simulink model "Bruening_4t_showshuffle"  (R2015a)
settings: Solver=ode4  SolverMode=MultiTasking  StartTime=0.0  StopTime=inf  FixedStep=BKIN_STEP_TIME  RelTol=1e-3
StartFcn:
  |  warndlg('Dexterit-E models cannot run under simulation. Please compile your model and run it from within Dexterit-E.');set_param(bdroot,'SimulationCommand','stop')
model workspace (MAT data in the model file):
  BKIN_STEP_TIME = 0.00025
  col_x = 1
  col_y = 2
  E_TARGET_ON = 3
  E_HOLD_AT_TARGET = 5
  LOGICAL_RADIUS = 4
  START_TARGET_COL = 1
  END_TARGET_COL = 2
  ROTATION_CENTER = 5
  WAIT_AT_1stTARGET_COL = 7
  MAXREACHTIME_COL = 8
  DELAY_POSTTRIAL_COL = 9
  E_STAY_CENTER = 2
  VISUAL_RADIUS = 3
  COLOR = 5
  ALTCOLOR = 6
  STROKECOLOUR = 7
  STROKEWIDTH = 9
  TARGET_EGG = 6
  LABEL_TEXT = 12
  LABEL_COLOUR = 13
  LABEL_HEIGHT = 14
  TEXT_DISPLAY_TARGET = 10
  ALTSTROKECOLOUR = 8
  SEGMENT_COUNT = 11
  E_TARGET_MISS = 6
  END_X = 10
  END_Y = 11
  E_LEFT_RING = 4
  E_START_BLOCK = 10
  BKIN_KINEMATIC_FRAME_SIZE = 400
  E_NO_EVENT = 1
  TARGET_IN_USE = 3
  R_PROB = 4
  E_R_TARG1 = 7
  E_M_TARG1 = 12
  E_R_TARG2 = 8
  E_M_TARG2 = 13
  E_R_TARG3 = 9
  E_M_TARG3 = 14
  E_R_TARG4 = 11
  E_M_TARG4 = 15
  WAIT_TIME = 12
  TONE_DURATION = 13
  FLASH_INTER = 14
  FLASH_NUM = 15
  BREAK_T1 = 16
  BREAK_T2 = 17
  ALTVISUAL_RADIUS = 15
  ALTCOLOR2 = 16
undefined symbols (not defined in the file or in its folder): slselsubs
libraries: Video x15, simulink x12, xpcrtudplib x12, xpcutilitieslib x10, xpcobsoletelib x8, ethercat x2, General x2, slrtlib x2, KINARM_general x1
(part 1 of 6)
CloseFcn:
  | rtwprivate ssgencode ModelCloseRequest b2lab2d
settings Model: ModifiedComment=chris -- Wed Feb 16 09:18:30 2005 -- Version 1.1384  ModifiedHistory=Feb 16/05 - Add error repeat, add offset ramp  CovHTMLOptions=-sRT=1 -sVT=0 -aTS=1 -bRG=1 -bTC=1 -hTR=0 -nFC=0 -scm=1 -bcm=1 -xEv=0  ExtModeArmWhenConnect=off  ExtModeLogAll=off  Creator=Chris Grebeldinger  LastModifiedBy=User
settings SolverCC: EnableConcurrentExecution=on  AutoInsertRateTranBlk=on
settings DataIOCC: LimitDataPoints=off  SignalLoggingSaveFormat=ModelDataLogs  SaveOutput=off  SaveTime=off  SignalLoggingName=sigsOut
settings OptimizationCC: BlockReduction=off  BooleanDataType=off  OptimizeBlockIOStorage=off  BufferReuse=off  GlobalBufferReuse=off  ExpressionFolding=off  ExpressionDepthLimit=2147483647  LocalBlockOutputs=off  InitFltsAndDblsToZero=on
settings DebuggingCC: SaveWithParameterizedLinksMsg=none  UnderspecifiedInitializationDetection=Classic  MergeDetectMultiDrivingBlocksExec=none  SignalResolutionControl=TryResolveAll  MultiTaskDSMMsg=warning  FcnCallInpInsideContextMsg=UseLocalSettings  StateNameClashWarn=warning  StrictBusMsg=ErrorOnBusTreatedAsVector
settings HardwareCC: ProdIntDivRoundTo=Zero  ProdEndianess=LittleEndian  ProdLongLongMode=on  ProdHWDeviceType=Generic->32-bit x86 compatible  TargetHWDeviceType=32-bit Generic
settings SFSimCC: SimParseCustomCode=off
settings RTWCC: SystemTargetFile=slrt.tlc  TemplateMakefile=slrt_default_tmf  Description=Simulink Real-Time  RTWCompilerOptimization=on
settings CodeAppCC: MaxIdLength=63
settings SimulinkRealTimeCC: TargetFcnLib=ansi_tfl_tmw.mat  GeneratePreprocessorConditionals=Disable all  xPCisDownloadable=off
settings ConfigComp: Description=Design Verifier Custom Configuration Component  DVMaxTestCaseSteps=500  DVTestSuiteOptimization=CombinedObjectives (Nonlinear Extended)

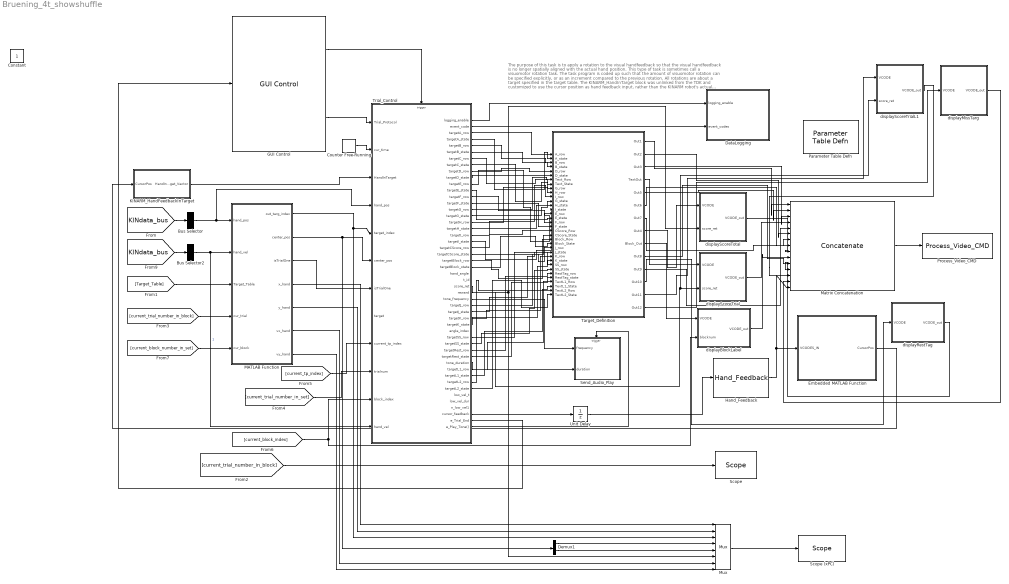
== system Bruening_4t_showshuffle ==
  note: The purpose of this task is to apply a rotation to the visual handfeedback so that the visual handfeedback is no longer spatially aligned with the actual hand position.
      | This type of task is sometimes call a visuomotor rotation task.
      | The task program is coded up such that the amount of visuomotor rotation can be specified explicitly, or as an increment compared to the previous rotation.
      | All rotations are about a target specified in the target table.
      |
      | The KINARM_HandInTarget block was unlinked from the TDK and customized to use the cursor position as hand feedback input, rather than the KINARM robot's actual location.
  Bus Selector : BusSelector  OutputSignals=Robot1.a1_hand_position  OutputAsBus=on
  Bus Selector2 : BusSelector  OutputSignals=Robot1.a1_hand_velocities  OutputAsBus=on
  Counter Free-Running : simulink/Sources/Counter Free-Running  NumBits=32  tsamp=.001
  DataLogging : Subsystem  AncestorBlock=General/DataLogging  mask(DataLogging){log_event_codes=on, log_analog_inputs=off}
      mask prompts: log_event_codes "Log event codes"; log_analog_inputs "Log analog inputs"
      mask help:
      | <b>Do not rename this block, it must be called 'DataLogging'.</b>
      | <p>
      | This block collects data and event codes and transfers them to the GUI.
      | <p>
      | This block must be present in all task programs.
      mask init:
      | %this stops us from running a simulation
      | set_param(bdroot,'StartFcn',' warndlg(''Dexterit-E models cannot run under simulation. Please compile your model and run it from within Dexterit-E.'');set_param(bdroot,''SimulationCommand'',''stop'')')
      | 
      | block_path = gcb;  % store block path, as gcb may change with block operations
      |  
      | idxs = findstr(block_path, '/DataLogging');
      | [idxCount, n] = size(idxs);
      | [m, strlen] = size(block_path);
      | bColorSet = 0;
      | 
      | dexcheck();
      | if idxCount == 0 || idxs(1) ~= strlen - 11
      |     fprintf('=========ERROR====================\n');
      |     fprintf('%s should be called DataLogging, attempting to rename.\n', block_path);
      |     try
      |         set_param(block_path, 'Name', 'DataLogging');
      |         block_path = gcb;  % store block path, as gcb may change with block operations
      |         fprintf('Rename successful\n');
      |     catch err
      |         fprintf('Rename failed. You may have 2 DataLogging blocks or another improperly named block.\n');
      |        	set_param(block_path, 'BackgroundColor', '[0.9, 0, 0]');
      |         bColorSet = 1;
      |     end
      |     fprintf('=============================\n');
      | end
      | 
      | log_event_codes = strcmp(get_param(block_path, 'log_event_codes'), 'on');
      | log_analog_inputs = strcmp(get_param(block_path, 'log_analog_inputs'), 'on');
      | 
      | % Handle the event codes setting: swap the 'Event Codes' inport with a constant block or 
      | % vice versa, if necessary, so that it matches the setting.
      | block_type = get_param([block_path '/event_codes'], 'BlockType');
      |  
      | if log_event_codes && ~strcmp(block_type, 'Inport') || ...  % if a change is required...
      |    ~log_event_codes && strcmp(block_type, 'Inport')
      |     
      |     % ...delete the existing block, ...
      |     pos = get_param([block_path '/event_codes'], 'Position');
      |     delete_line(block_path, 'event_codes/1', 'Create Event Codes Subsystem/1');
      |     delete_block([block_path '/event_codes']);
      |     
      |     % ...add an Inport or a 0-value Constant in place of the previous block (according to
      |     % the new setting), update the signal width flag, and then...
      |     if log_event_codes && ~strcmp(block_type, 'Inport')
      |         add_block('built-in/Inport', [block_path '/event_codes'], 'Name', 'event_codes');
      |         set_param([block_path '/Create Event Codes Subsystem/Not Logging Event Codes'], 'Value', '0');
      |     else
      |         add_block('built-in/Constant', [block_path '/event_codes'], 'Name', 'event_codes');
      |         set_param([block_path '/event_codes'], 'Value', '0');
      |         set_param([block_path '/Create Event Codes Subsystem/Not Logging Event Codes'], 'Value', '1');
      |     end
      |     
      |     % ...connect the new block.
      |     set_param([block_path '/event_codes'], 'Position', pos);
      |     add_line(block_path, 'event_codes/1', 'Create Event Codes Subsystem/1');
      | end
      | 
      | % Swap the 'analog_data' inport with a constant block or vice versa according to the corresponding setting.
      | block_type = get_param([block_path '/analog_inputs'], 'BlockType');
      | 
      | if log_analog_inputs && ~strcmp(block_type, 'Inport') || ...  % if a change is required...
      |    ~log_analog_inputs && strcmp(block_type, 'Inport')
      |     
      |     % ...delete the existing block, ...
      |     pos = get_param([block_path '/analog_inputs'], 'Position');
      |     delete_line(block_path, 'analog_inputs/1', 'Create Analog Inputs Subsystem/1');
      |     delete_block([block_path '/analog_inputs']);
      |     
      |     % ...add an Inport or a 0-value Constant in place of the previous block (according to
      |     % the new setting), update the signal width flag, and then...
      |     if log_analog_inputs && ~strcmp(block_type, 'Inport')
      |         add_block('built-in/Inport', [block_path '/analog_inputs'], 'Name', 'analog_inputs');
      |         set_param([block_path '/Create Analog Inputs Subsystem/Not Logging Analog Inputs'], 'Value', '0');
      |     else
      |         add_block('built-in/Constant', [block_path '/analog_inputs'], 'Name', 'analog_inputs');
      |         set_param([block_path '/analog_inputs'], 'Value', '0');
      |         set_param([block_path '/Create Analog Inputs Subsystem/Not Logging Analog Inputs'], 'Value', '1');
      |     end
      |     
      |     % ...connect the new block.
      |     set_param([block_path '/analog_inputs'], 'Position', pos);
      |     add_line(block_path, 'analog_inputs/1', 'Create Analog Inputs Subsystem/1');
      | end
      | 
      | % Create the text label for the block, and use it to create the first in a 
      | % list of drawing commands that will be used to draw the mask icon.
      | label = 'Logging:\n ';
      |  
      | if log_event_codes
      |    label = [label 'Event codes\n'];
      | end
      |  
      | label = [label 'KINARM data\n'];
      |     
      | if log_analog_inputs
      |     label = [label 'Analog inputs\n'];
      | end
      | 
      | draw_commands = 'disp(label); ';
      | 
      | % Ensure the inports appear in a fixed order, and for each inport found add
      | % to the list of drawing commands a command to label it.
      | inports = find_system(block_path, 'LookUnderMasks', 'all', 'FollowLinks', 'on', 'SearchDepth', 1, 'BlockType', 'Inport');
      | 
      | for i = 1:length(inports)
      |     inport_name = char(get_param(inports(i), 'Name'));
      |     
      |     if strcmp(inport_name, 'logging_enable')
      |         port = '1';
      |     elseif strcmp(inport_name, 'event_codes')
      |         port = '2';
      |     elseif strcmp(inport_name, 'analog_inputs') && log_event_codes
      |         port = '3';
      |     elseif strcmp(inport_name, 'analog_inputs')
      |         port = '2';
      |     end
      |     
      |     set_param([block_path '/' inport_name], 'Port', port);
      |     draw_commands = [draw_commands 'port_label(''input'', ' port ', ''' inport_name '''); '];
      | end
      | 
      | % Apply the drawing commands.
      | set_param(block_path, 'MaskDisplay', draw_commands);
      | 
      | %%% Handle background colours if link status changes.  
      | checkBackgroundColour(block_path, 'General');
      | 
      | % For gaze tracking, the packet length is variable, so we need to check off that option the Receive UDP block.
      | set_param([block_path '/Receive_Gaze/Receive'], 'vblLen', 'on')
      | 
      | initPollKINARM();
      mask Help:
      | Sends data and event codes to the GUI.
      | 
      | <H2>Library </H2>
      | General
      | 
      | <H2>Description </H2>
      | <b>Do not rename this block, it must be called 'DataLogging'.</b>
      | <p>
      | The DataLogging block collects data and event codes and sends it to the GUI for saving.  It also passes on Task Program information that is invisible to the user, and so must be present even if no data is going to be saved.
      | <P>
      | <B><I>This block must be present in all Task Programs, even if no data is going to be saved.</I></B>
      | 
      | 
      | <H2>Parameters and Dialog Box</H2>
      | <B>Log event codes: </B> checking this parameter causes the GUI to log event codes specified by the event_codes input.
      | <P>
      | <B>Log analog inputs: </B> checking this parameter causes the GUI to log analog data specified by the analog_inputs input.
      | <P>
      | <B>analog_inputs: </B> this vector input specifies the data from analog inputs and other arbitrary data to be logged by the GUI.
      | <P>
      | <B>event_codes: </B> this input should be a vector of 16 bit integers.  It is passed on to the GUI, which saves the integers as event codes (i.e. they are timestamped so that events that occurred duing a task can be related to the other saved data).
      | <P>
      | <B>logging_enable: </B> this input is used by the GUI to indicate when to save data.  When logging_enable is 1, data is saved.  When logging_enable is 0, data is not saved.  (Note: data saving is also affected by the Run/Pause button in the GUI.  When the task is paused, data is no longer saved regardless of the value of this input).
      mask Display: disp(label); port_label('input', 1, 'logging_enable'); port_label('input', 2, 'event_codes');
  Demux1 : Demux  Outputs=2
  Embedded MATLAB Function : MATLAB Function  TreatAsAtomicUnit=on
  GUI Control : General/GUI Control  target_type_str=Circle  Target_Type=1  XYcols=[1 2]  Vcols=3  Lcols=4  indices_padding=[0 0 0 0;0 0 0 0]  task_version=1.0  show_repeat_trial_flag=off
  Hand_Feedback : KINARM_general/Hand_Feedback  feedback_cntl_src=status only
  KINARM_HandFeedbackInTarget : Subsystem  AncestorBlock=KINARM_general/KINARM_HandInTarget  mask(KINARM_HandInTarget){use_dominant_hand=on, target_type=Circle, num_states=1, attribcol1=4, attribcol2=3, attribcol3=3, attribcol4=3}
      mask prompts: use_dominant_hand "Dominant Hand?"; target_type "Type of Target"; num_states "Number of Target States"; attribcol1 "State 1 Target Table Column(s)"; attribcol2 "State 2 Target Table Column(s)"; attribcol3 "State 3 Target Table Column(s)"; attribcol4 "State 4 Target Table Column(s)"
      mask help: This block returns a vector or array corresponding to the Target_Table rows indicating whether the specified hand is in (=1) or out (=0) of each of the targets.
      mask init:
      | num_states=str2num(get_param(gcb, 'num_states'));
      | columntext='(columns: ';
      | 
      | for i=1:num_states
      | 	varname=['attribcol' num2str(i)];
      | 	if i>1
      | 		columntext=[columntext, '; '];
      | 	end
      | 	columntext=[columntext, get_param(gcb, varname)];
      | end
      | columntext=strvcat([columntext ')'],' ', ' ');
      | 
      | output_block=char(find_system(gcb,'LookUnderMasks','all','FollowLinks','on','SearchDepth',1,'BlockType','Outport'));
      | outputname=get_param(output_block,'Name');
      | 
      | % Select only the desired states for output. The output port is also renamed to reflect 
      | % whether the output is a vector (in the case of a single state) or an array (of vectors, 
      | % one for each of multiple states).
      | if num_states == 1
      | 	set_param([gcb '/Selected States'], 'Value', '[1]');
      | 	set_param(output_block, 'Name', 'HandInTarget_Vector');
      | elseif num_states == 2
      | 	set_param([gcb '/Selected States'], 'Value', '[1,2]');
      | 	set_param(output_block, 'Name', 'HandInTarget_Array');
      | elseif num_states == 3
      | 	set_param([gcb '/Selected States'], 'Value', '[1,2,3]');
      | 	set_param(output_block, 'Name', 'HandInTarget_Array');
      | else
      | 	set_param([gcb '/Selected States'], 'Value', '[1,2,3,4]');
      | 	set_param(output_block, 'Name', 'HandInTarget_Array');
      | end
      mask Help:
      | Used to determine if the hand (finger-tip) is in any of the targets in the Target_Table.
      | <P>
      | <B><I>Use of this block requires that the DataLogging block (General library) be set to log KINARM data.</I></B>
      | 
      | <H2>Library </H2>
      | KINARM_general (sub-library)
      | 
      | <H2>Description </H2>
      | This block returns a vector or array corresponding to the Target_Table rows indicating whether the specified hand (i.e. finger-tip) is in or out of each of the targets.  Each element in the output vector or output array will be either a 0 (hand not in target) or a 1 (hand in target).
      | <P>
      | A vector is returned if only one target state is specified in each target row (see Parameters and Dialog Box), with each index of the vector corresponding to a row in the target table.  An array is returned if more than one target state is specified in a target row, with each row of the array corresponding to a target row and each column corresponding to the nth target state specified in each target row.
      | <P>
      | The output vector or array is typically used by a stateflow chart to affect behavior of the system.  Because this block returns hand-in-target information for all targets in the target table, multiple targets can be monitored at once (i.e. the stateflow chart could have certain transitions that occur if the hand is in one target and other transitions if it is in a different target).  Likewise, because this block returns hand-in-target information for multiple states of a single target, those multiple states can be monitored simultaneously.
      | <P>
      | Because the KINARM_HandInTarget block returns information for only one hand, two copies of this block are required if information for both hands is desired.
      | <P>
      | 
      | <H2>Parameters and Dialog Box</H2>
      | <B>Dominant Hand?:</B> this box determines which hand is used by this block : dominant hand position (checked box) or the non-dominant hand position (unchecked box).  (Note: if the end-user wants to know about both the dominant hand and the non-dominant hand, then 2 separate copies of this block are requried, one for each hand.)
      | <P>
      | <B>Type of Target:</B> Enter the type of target specified in the target table:
      | <P>
      | <B>Number of Target States:</B> Enter the number of target states specified in each target row.  Up to four target states are allowed per target row.
      | <P>
      | <B>State <n> Target Table Columns:</B> Enter the columns in the Target Table that specify the relevant target attributes.  Do this for each target state.
      | For a circle, enter the columns corresponding to logical radius (e.g. 4)
      | <BR>For an ellipse, enter the columns corresponding to major radius, minor radius, rotation angle (e.g. [4, 5, 6]).
      | <BR>For a rectangle, enter the columns corresponding to length, height, and rotation angle (e.g. [4, 5, 6]).
      | <BR>For a line, enter the columns corresponding to stroke width, endpoint in x, and endpoint in y (e.g. [3, 4, 5]).
      | <BR>For a triangle, enter the columns corresponding to length, height, peak offset, and rotation angle (e.g. [4, 5, 6, 7]).
      | 
      | <H2>Examples</H2>
      | <B>Example 1.</B>  Suppose a target row will be used to define 1 state for a circle type target and the radius of the visual target is the same radius to be used for determination of hand-in-target.  The related Target Table column is: column 6 = radius.  For this example, "State 1 Target Table Columns" would equal [6].
      | <P>
      | 
      | <B>Example 2.</B>  Suppose a target row will be used to define 1 state for a circle type target, but the radius of the visual target will be different than the radius to be used for determination of hand-in-target.  This option allows independent control over the size of the visual target versus the accuracy needed to be considered "in the target".  The related Target Table columns are: column 6 = radius1 (i.e. radius to target to be drawn); column 7 = radius2 (i.e. radius to be used for hand-in-target) .  For this example, "State 1 Target Table Columns" would equal [7].
      | <P>
      | <B>Example 3.</B>  Suppose a target row will be used to define 2 states for a circle type target, where the radius of the visual target will be a constant, but depending on the state of the system, one of 2 other and different radii will be used for determination of hand-in-target.  The related Target Table columns are: column 6 = radius1 (i.e. radius to target to be drawn); column 7 = radius2 (i.e. radius to be used for hand-in-target for state 1); column 8 = radius3 (i.e. radius to be used for hand-in-target for state 2).  For this example, "State 1 Target Table Columns" would equal [7], while "State 2 Target Table Columns" would equal [8].
      | <P>
      | 
      | <H2>Related Blocks </H2>
      | DataLogging
      mask TypeOptions target_type: Circle | Ellipse | Rectangle | Line | Triangle
      mask Callback target_type:
      | target_type=get_param(gcb, 'target_type');
      | attribcol1=[str2num(get_param(gcb, 'attribcol1')) 0 0 0 0 0 0];
      | attribcol2=[str2num(get_param(gcb, 'attribcol2')) 0 0 0 0 0 0];
      | attribcol3=[str2num(get_param(gcb, 'attribcol3')) 0 0 0 0 0 0];
      | attribcol4=[str2num(get_param(gcb, 'attribcol4')) 0 0 0 0 0 0];
      | switch target_type(1:3)
      | 	case 'Cir'
      | 		numcol=1;
      | 	case 'Ell'
      | 		numcol=3;
      |     case 'Rec'
      |         numcol=3;
      |     case 'Lin'
      |         numcol=3;
      |     case 'Tri'
      |         numcol=4;
      | 	otherwise
      | 		numcol=1;
      | end
      | if numcol==1
      | 	set_param(gcb, 'attribcol1', num2str(attribcol1(1)));
      | 	set_param(gcb, 'attribcol2', num2str(attribcol2(1)));
      | 	set_param(gcb, 'attribcol3', num2str(attribcol3(1)));
      | 	set_param(gcb, 'attribcol4', num2str(attribcol4(1)));
      | else
      | 	set_param(gcb, 'attribcol1', ['[' num2str(attribcol1(1:numcol)) ']']);
      | 	set_param(gcb, 'attribcol2', ['[' num2str(attribcol2(1:numcol)) ']']);
      | 	set_param(gcb, 'attribcol3', ['[' num2str(attribcol3(1:numcol)) ']']);
      | 	set_param(gcb, 'attribcol4', ['[' num2str(attribcol4(1:numcol)) ']']);
      | end
      mask TypeOptions num_states: 1 | 2 | 3 | 4
      mask Callback num_states:
      | num_states = str2num(get_param(gcb, 'num_states'));
      | vis = get_param(gcb, 'MaskVisibilities');
      | 
      | % Select only the desired states for output. The output port is also renamed to reflect
      | % whether the output is a vector (in the case of a single state) or an array (of vectors,
      | % one for each of multiple states).
      | output_block=char(find_system(gcb, 'LookUnderMasks', 'all', 'FollowLinks', 'on', 'SearchDepth', 1, 'BlockType', 'Outport'));
      | 
      | if num_states == 1
      | 	set_param([gcb '/Selected States'], 'Value', '[1]');
      | 	set_param(output_block, 'Name', 'HandInTarget_Vector');
      | 	vis{5} = 'off';
      | 	vis{6} = 'off';
      | 	vis{7} = 'off';
      | elseif num_states == 2
      | 	set_param([gcb '/Selected States'], 'Value', '[1,2]');
      | 	set_param(output_block, 'Name', 'HandInTarget_Array');
      | 	vis{5} = 'on';
      | 	vis{6} = 'off';
      | 	vis{7} = 'off';
      | elseif num_states == 3
      | 	set_param([gcb '/Selected States'], 'Value', '[1,2,3]');
      | 	set_param(output_block, 'Name','HandInTarget_Array');
      | 	vis{5} = 'on';
      | 	vis{6} = 'on';
      | 	vis{7} = 'off';
      | else
      | 	set_param([gcb '/Selected States'], 'Value', '[1,2,3,4]');
      | 	set_param(output_block, 'Name', 'HandInTarget_Array');
      | 	vis{5} = 'on';
      | 	vis{6} = 'on';
      | 	vis{7} = 'on';
      | end
      | set_param(gcb, 'MaskVisibilities', vis);
      | 
      | target_type=get_param(gcb, 'target_type');
      | attribcol1=[str2num(get_param(gcb, 'attribcol1')) 0 0 0 0 0 0];
      | attribcol2=[str2num(get_param(gcb, 'attribcol2')) 0 0 0 0 0 0];
      | attribcol3=[str2num(get_param(gcb, 'attribcol3')) 0 0 0 0 0 0];
      | attribcol4=[str2num(get_param(gcb, 'attribcol4')) 0 0 0 0 0 0];
      | switch target_type(1:3)
      | 	case 'Cir'
      | 		numcol=1;
      | 	case 'Ell'
      | 		numcol=3;
      |     case 'Rec'
      |         numcol=3;
      |     case 'Lin'
      |         numcol=3;
      |     case 'Tri'
      |         numcol=4;
      | 	otherwise
      | 		numcol=1;
      | end
      | if numcol==1
      | 	set_param(gcb, 'attribcol1', num2str(attribcol1(1)));
      | 	set_param(gcb, 'attribcol2', num2str(attribcol2(1)));
      | 	set_param(gcb, 'attribcol3', num2str(attribcol3(1)));
      | 	set_param(gcb, 'attribcol4', num2str(attribcol4(1)));
      | else
      | 	set_param(gcb, 'attribcol1', ['[' num2str(attribcol1(1:numcol)) ']']);
      | 	set_param(gcb, 'attribcol2', ['[' num2str(attribcol2(1:numcol)) ']']);
      | 	set_param(gcb, 'attribcol3', ['[' num2str(attribcol3(1:numcol)) ']']);
      | 	set_param(gcb, 'attribcol4', ['[' num2str(attribcol4(1:numcol)) ']']);
      | end
      mask Callback attribcol1:
      | target_type=get_param(gcb, 'target_type');
      | attribcol1=[str2num(get_param(gcb, 'attribcol1')) 0 0 0 0 0 0];
      | attribcol2=[str2num(get_param(gcb, 'attribcol2')) 0 0 0 0 0 0];
      | attribcol3=[str2num(get_param(gcb, 'attribcol3')) 0 0 0 0 0 0];
      | attribcol4=[str2num(get_param(gcb, 'attribcol4')) 0 0 0 0 0 0];
      | switch target_type(1:3)
      | 	case 'Cir'
      | 		numcol=1;
      | 	case 'Ell'
      | 		numcol=3;
      |     case 'Rec'
      |         numcol=3;
      |     case 'Lin'
      |         numcol=3;
      |     case 'Tri'
      |         numcol=4;
      | 	otherwise
      | 		numcol=1;
      | end
      | if numcol==1
      | 	set_param(gcb, 'attribcol1', num2str(attribcol1(1)));
      | 	set_param(gcb, 'attribcol2', num2str(attribcol2(1)));
      | 	set_param(gcb, 'attribcol3', num2str(attribcol3(1)));
      | 	set_param(gcb, 'attribcol4', num2str(attribcol4(1)));
      | else
      | 	set_param(gcb, 'attribcol1', ['[' num2str(attribcol1(1:numcol)) ']']);
      | 	set_param(gcb, 'attribcol2', ['[' num2str(attribcol2(1:numcol)) ']']);
      | 	set_param(gcb, 'attribcol3', ['[' num2str(attribcol3(1:numcol)) ']']);
      | 	set_param(gcb, 'attribcol4', ['[' num2str(attribcol4(1:numcol)) ']']);
      | end
      mask Callback attribcol2:
      | target_type=get_param(gcb, 'target_type');
      | attribcol1=[str2num(get_param(gcb, 'attribcol1')) 0 0 0 0 0 0];
      | attribcol2=[str2num(get_param(gcb, 'attribcol2')) 0 0 0 0 0 0];
      | attribcol3=[str2num(get_param(gcb, 'attribcol3')) 0 0 0 0 0 0];
      | attribcol4=[str2num(get_param(gcb, 'attribcol4')) 0 0 0 0 0 0];
      | switch target_type(1:3)
      | 	case 'Cir'
      | 		numcol=1;
      | 	case 'Ell'
      | 		numcol=3;
      |     case 'Rec'
      |         numcol=3;
      |     case 'Lin'
      |         numcol=3;
      |     case 'Tri'
      |         numcol=4;
      | 	otherwise
      | 		numcol=1;
      | end
      | if numcol==1
      | 	set_param(gcb, 'attribcol1', num2str(attribcol1(1)));
      | 	set_param(gcb, 'attribcol2', num2str(attribcol2(1)));
      | 	set_param(gcb, 'attribcol3', num2str(attribcol3(1)));
      | 	set_param(gcb, 'attribcol4', num2str(attribcol4(1)));
      | else
      | 	set_param(gcb, 'attribcol1', ['[' num2str(attribcol1(1:numcol)) ']']);
      | 	set_param(gcb, 'attribcol2', ['[' num2str(attribcol2(1:numcol)) ']']);
      | 	set_param(gcb, 'attribcol3', ['[' num2str(attribcol3(1:numcol)) ']']);
      | 	set_param(gcb, 'attribcol4', ['[' num2str(attribcol4(1:numcol)) ']']);
      | end
      mask Callback attribcol3:
      | target_type=get_param(gcb, 'target_type');
      | attribcol1=[str2num(get_param(gcb, 'attribcol1')) 0 0 0 0 0 0];
      | attribcol2=[str2num(get_param(gcb, 'attribcol2')) 0 0 0 0 0 0];
      | attribcol3=[str2num(get_param(gcb, 'attribcol3')) 0 0 0 0 0 0];
      | attribcol4=[str2num(get_param(gcb, 'attribcol4')) 0 0 0 0 0 0];
      | switch target_type(1:3)
      | 	case 'Cir'
      | 		numcol=1;
      | 	case 'Ell'
      | 		numcol=3;
      |     case 'Rec'
      |         numcol=3;
      |     case 'Lin'
      |         numcol=3;
      |     case 'Tri'
      |         numcol=4;
      | 	otherwise
      | 		numcol=1;
      | end
      | if numcol==1
      | 	set_param(gcb, 'attribcol1', num2str(attribcol1(1)));
      | 	set_param(gcb, 'attribcol2', num2str(attribcol2(1)));
      | 	set_param(gcb, 'attribcol3', num2str(attribcol3(1)));
      | 	set_param(gcb, 'attribcol4', num2str(attribcol4(1)));
      | else
      | 	set_param(gcb, 'attribcol1', ['[' num2str(attribcol1(1:numcol)) ']']);
      | 	set_param(gcb, 'attribcol2', ['[' num2str(attribcol2(1:numcol)) ']']);
      | 	set_param(gcb, 'attribcol3', ['[' num2str(attribcol3(1:numcol)) ']']);
      | 	set_param(gcb, 'attribcol4', ['[' num2str(attribcol4(1:numcol)) ']']);
      | end
      mask Callback attribcol4:
      | target_type=get_param(gcb, 'target_type');
      | attribcol1=[str2num(get_param(gcb, 'attribcol1')) 0 0 0 0 0 0];
      | attribcol2=[str2num(get_param(gcb, 'attribcol2')) 0 0 0 0 0 0];
      | attribcol3=[str2num(get_param(gcb, 'attribcol3')) 0 0 0 0 0 0];
      | attribcol4=[str2num(get_param(gcb, 'attribcol4')) 0 0 0 0 0 0];
      | switch target_type(1:3)
      | 	case 'Cir'
      | 		numcol=1;
      | 	case 'Ell'
      | 		numcol=3;
      |     case 'Rec'
      |         numcol=3;
      |     case 'Lin'
      |         numcol=3;
      |     case 'Tri'
      |         numcol=4;
      | 	otherwise
      | 		numcol=1;
      | end
      | if numcol==1
      | 	set_param(gcb, 'attribcol1', num2str(attribcol1(1)));
      | 	set_param(gcb, 'attribcol2', num2str(attribcol2(1)));
      | 	set_param(gcb, 'attribcol3', num2str(attribcol3(1)));
      | 	set_param(gcb, 'attribcol4', num2str(attribcol4(1)));
      | else
      | 	set_param(gcb, 'attribcol1', ['[' num2str(attribcol1(1:numcol)) ']']);
      | 	set_param(gcb, 'attribcol2', ['[' num2str(attribcol2(1:numcol)) ']']);
      | 	set_param(gcb, 'attribcol3', ['[' num2str(attribcol3(1:numcol)) ']']);
      | 	set_param(gcb, 'attribcol4', ['[' num2str(attribcol4(1:numcol)) ']']);
      | end
      mask Display:
      | disp(columntext)
      | port_label('output',1,outputname)
  MATLAB Function : MATLAB Function  TreatAsAtomicUnit=on
  Matrix Concatenation : Concatenate  NumInputs=15  Mode=Multidimensional array
  Mux : Mux  Inputs=8
  Parameter Table Defn : General/Parameter Table Defn  ShowInLibBrowser=0
  Process_Video_CMD : Video/Process_Video_CMD
  "Scope " : slrtlib/Displays and Logging/Scope   scopeno=2  scopetype=Target  autostart=on  viewmode=Numerical  formatstr='%15.6f'  grid=on  ylimits=[0,0]  nosamples=250  noprepostsamples=0  interleave=1  triggermode=FreeRun  triggersignal=1  trigsignalfromport=off  triggerlevel=0.0  triggerslope=Either  triggerscope=1  triggersample=0  filename=data.dat  mode=Lazy  writesize=512  autorestart=off  dynamicfilemode=off  maxwritefilesize=512*1024^2
  "Scope (xPC) " : slrtlib/Displays and Logging/Scope   scopeno=1  scopetype=Target  autostart=on  viewmode=Numerical  formatstr='%15.6f'  grid=on  ylimits=[0,0]  nosamples=250  noprepostsamples=0  interleave=1  triggermode=FreeRun  triggersignal=1  trigsignalfromport=off  triggerlevel=0.0  triggerslope=Either  triggerscope=1  triggersample=0  filename=data.dat  mode=Lazy  writesize=512  autorestart=off  dynamicfilemode=off  maxwritefilesize=512*1024^2
  Send_Audio_Play : Subsystem  AncestorBlock=General/DataLogging/Network Transfer Subsystem/UDP Send Subsystem  TreatAsAtomicUnit=on
  "Target_Definition " : Subsystem
  Trial_Control : Stateflow chart  TreatAsAtomicUnit=on
  Unit Delay : UnitDelay  SampleTime=-1
  displayBlockLabel : MATLAB Function  TreatAsAtomicUnit=on
  displayMissTarg : MATLAB Function  TreatAsAtomicUnit=on
  displayRestTag : MATLAB Function  TreatAsAtomicUnit=on
  displayScoreTotal : MATLAB Function  TreatAsAtomicUnit=on
  displayScoreTrial : MATLAB Function  TreatAsAtomicUnit=on
  displayScoreTrialL1 : MATLAB Function  TreatAsAtomicUnit=on
  Constant : Constant  IOType=siggen
  wires:
  GUI Control/2 -> Trial_Control/1(Trial_Protocol)
  GUI Control/1 -> Trial_Control/Trigger
  Trial_Control/2(event_code) -> DataLogging/2(event_codes)
  Matrix Concatenation/1 -> Process_Video_CMD/1
  KINARM_HandFeedbackInTarget/1(HandInTarget_Vector) -> Trial_Control/3(HandInTarget)
  Trial_Control/1(logging_enable) -> DataLogging/1(logging_enable)
  Hand_Feedback/1 -> Matrix Concatenation/15, Embedded MATLAB Function/1(VCODES_IN)
  Embedded MATLAB Function/1(CursorPos) -> KINARM_HandFeedbackInTarget/1(CursorPos)
  [KINdata_bus] -> Bus Selector/1
  [Target_Table] -> MATLAB Function/3(Target_Table)
  Bus Selector/1 -> Trial_Control/4(hand_pos), MATLAB Function/1(hand_pos)
  MATLAB Function/1(out_targ_index) -> Trial_Control/5(target_index), Mux/3
  Trial_Control/48(e_Trial_End) -> GUI Control/1
  displayScoreTrial/1(VCODE_out) -> Matrix Concatenation/4
  Mux/1 -> "Scope (xPC) "/1
  MATLAB Function/4(x_hand) -> Mux/1
  MATLAB Function/5(y_hand) -> Mux/2
  MATLAB Function/2(center_pos) -> Demux1/1, Trial_Control/6(center_pos)
  "Target_Definition "/1(Out1) -> Matrix Concatenation/1
  "Target_Definition "/3(Out3) -> Matrix Concatenation/3
  "Target_Definition "/4(TextOut) -> displayScoreTrial/1(VCODE)
  [current_trial_number_in_block] -> "Scope "/1
  Demux1/2 -> Mux/5
  Demux1/1 -> Mux/4
  "Target_Definition "/6(Out6) -> Matrix Concatenation/7
  "Target_Definition "/7(Out7) -> Matrix Concatenation/8
  Trial_Control/3(targetA_row) -> "Target_Definition "/1(A_row)
  Trial_Control/4(targetA_state) -> "Target_Definition "/2(A_state)
  Trial_Control/5(targetB_row) -> "Target_Definition "/3(B_row)
  Trial_Control/6(targetB_state) -> "Target_Definition "/4(B_state)
  Trial_Control/9(targetD_row) -> "Target_Definition "/5(D_row)
  Trial_Control/10(targetD_state) -> "Target_Definition "/6(D_state)
  Trial_Control/7(targetC_row) -> "Target_Definition "/7(Text_Row)
  Trial_Control/8(targetC_state) -> "Target_Definition "/8(Text_State)
  Trial_Control/11(targetE_row) -> "Target_Definition "/15(E_row)
  Trial_Control/12(targetE_state) -> "Target_Definition "/16(E_state)
  Trial_Control/13(targetF_row) -> "Target_Definition "/17(F_row)
  Trial_Control/14(targetF_state) -> "Target_Definition "/18(F_state)
  Trial_Control/16(targetG_state) -> "Target_Definition "/12(G_state)
  Trial_Control/18(targetH_state) -> "Target_Definition "/13(H_state)
  Trial_Control/20(targetI_state) -> "Target_Definition "/14(I_state)
  Trial_Control/19(targetI_row) -> "Target_Definition "/11(I_row)
  Trial_Control/17(targetH_row) -> "Target_Definition "/10(H_row)
  Trial_Control/15(targetG_row) -> "Target_Definition "/9(G_row)
  MATLAB Function/3(isTrialOne) -> Trial_Control/7(isTrialOne)
  [current_trial_number_in_block] -> MATLAB Function/4(cur_trial)
  Trial_Control/28(reward) -> displayScoreTrialL1/2(score_ret), displayScoreTrial/2(score_ret)
  Trial_Control/27(score_ret) -> Mux/6, displayScoreTotal/2(score_ret)
  "Target_Definition "/8(Out4) -> displayScoreTotal/1(VCODE)
  displayScoreTotal/1(VCODE_out) -> Matrix Concatenation/9
  Trial_Control/21(targetCScore_row) -> "Target_Definition "/19(CScore_Row)
  Trial_Control/22(targetCScore_state) -> "Target_Definition "/20(CScore_State)
  Trial_Control/49(e_Play_Tone()) -> Send_Audio_Play/Trigger
  Trial_Control/29(tone_frequency) -> Send_Audio_Play/1(frequency)
  Trial_Control/23(targetBlock_row) -> "Target_Definition "/21(Block_Row)
  Trial_Control/24(targetBlock_state) -> "Target_Definition "/22(Block_State)
  "Target_Definition "/9(Block_Out) -> displayBlockLabel/1(VCODE)
  displayBlockLabel/1(VCODE_out) -> Matrix Concatenation/10
  Trial_Control/30(targetJ_row) -> "Target_Definition "/23(J_row)
  Trial_Control/31(targetJ_state) -> "Target_Definition "/24(J_state)
  Trial_Control/32(targetK_row) -> "Target_Definition "/25(K_row)
  Trial_Control/33(targetK_state) -> "Target_Definition "/26(K_state)
  "Target_Definition "/10(Out8) -> Matrix Concatenation/11
  [current_tp_index] -> Trial_Control/9(current_tp_index)
  Trial_Control/35(targetSS_row) -> "Target_Definition "/27(SS_row)
  Trial_Control/36(targetSS_state) -> "Target_Definition "/28(SS_state)
  "Target_Definition "/11(Out9) -> Matrix Concatenation/5
  [current_block_index] -> displayBlockLabel/2(blocknum), Trial_Control/11(block_index)
  "Target_Definition "/12(Out10) -> displayRestTag/1(VCODE)
  displayRestTag/1(VCODE_out) -> Matrix Concatenation/12
  Trial_Control/37(targetRest_row) -> "Target_Definition "/29(RestTag_row)
  Trial_Control/38(targetRest_state) -> "Target_Definition "/30(RestTag_state)
  Trial_Control/39(tone_duration) -> Send_Audio_Play/2(duration)
  [current_trial_number_in_set] -> Trial_Control/10(trialnum)
  Trial_Control/40(targetL1_row) -> "Target_Definition "/31(TextL1_Row)
  Trial_Control/41(targetL1_state) -> "Target_Definition "/32(TextL1_State)
  Trial_Control/42(targetL2_row) -> "Target_Definition "/33(TextL2_Row)
  Trial_Control/43(targetL2_state) -> "Target_Definition "/34(TextL2_State)
  "Target_Definition "/13(Out11) -> displayScoreTrialL1/1(VCODE)
  "Target_Definition "/14(Out12) -> displayMissTarg/1(VCODE)
  displayScoreTrialL1/1(VCODE_out) -> Matrix Concatenation/13
  displayMissTarg/1(VCODE_out) -> Matrix Concatenation/14
  [current_block_number_in_set] -> MATLAB Function/5(cur_block)
  "Target_Definition "/2(Out2) -> Matrix Concatenation/6
  "Target_Definition "/5(Out5) -> Matrix Concatenation/2
  [KINdata_bus] -> Bus Selector2/1
  MATLAB Function/6(vx_hand) -> Mux/7
  MATLAB Function/7(vy_hand) -> Mux/8
  Bus Selector2/1 -> Trial_Control/12(hand_vel), MATLAB Function/2(hand_vel)  "]"
  Counter Free-Running/1 -> Trial_Control/2(cur_time)
  Trial_Control/47(cursor_feedback) -> Unit Delay/1
  Unit Delay/1 -> Hand_Feedback/1

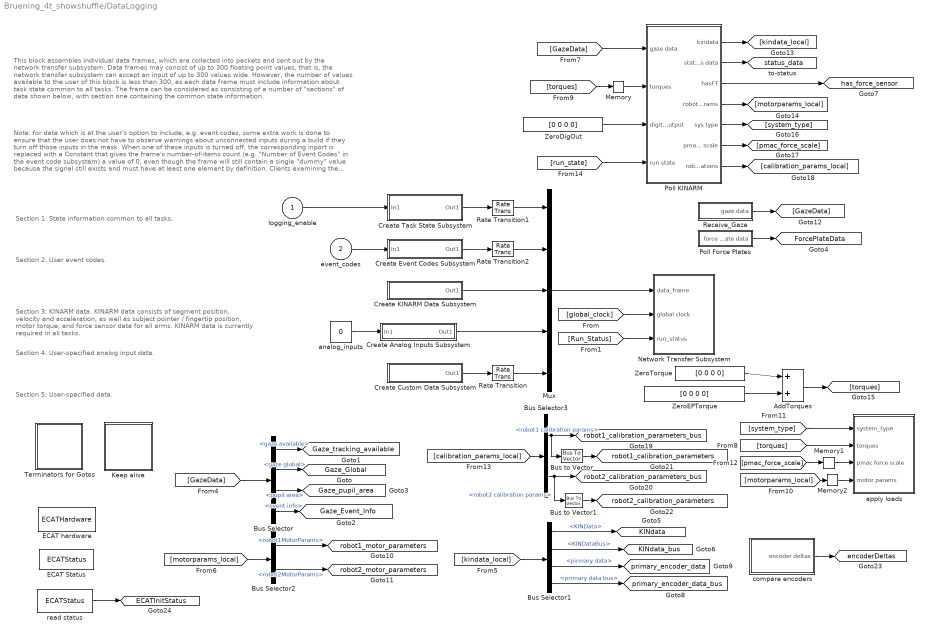
== system Bruening_4t_showshuffle/DataLogging ==
  note: Section 5: User-specified data.
  note: Note: for data which is at the user's option to include, e.g. event codes, some extra work is done to ensure that the user
      | does not have to observe warnings about unconnected inputs during a build if they turn off those inputs in the mask. When
      | one of these inputs is turned off, the corresponding inport is replaced with a Constant that gives the frame's number-of-items
      | count (e.g. "Number of Event Codes" in the event code subsystem) a value of 0, even though the frame will still contain a
      | single "dummy" value because the signal still exists and must have at least one element by definition. Clients examining the
      | data frames must be aware of this and ignore the dummy value.
      |
      | If a user opts to keep the inport available but connects nothing to it, Simulink resolves that as a single signal with value 0.
  note: Section 3: KINARM data. KINARM data consists of segment
      | position, velocity and acceleration, as well as subject pointer /
      | fingertip position, motor torque, and force sensor data for all arms.
      | KINARM data is currently required in all tasks.
  note: Section 2: User event codes.
  note: Section 1: State information common to all tasks.
  note: Section 4: User-specified analog input data.
  note: This block assembles individual data frames, which are collected into packets and sent out by the network transfer subsystem.
      |
      | Data frames may consist of up to 300 floating point values, that is, the network transfer subsystem can accept an input of up
      | to 300 values wide. However, the number of values available to the user of this block is less than 300, as each data frame
      | must include information about task state common to all tasks. The frame can be considered as consisting of a number of
      | "sections" of data shown below, with section one containing the common state information.
  logging_enable : Inport
  event_codes : Inport  Port=2
  AddTorques : Sum
  Bus Selector : BusSelector  OutputSignals=gaze available,gaze global,pupil area,event info
  Bus Selector1 : BusSelector  OutputSignals=KINData,KINDataBus,pirmary data,primary data bus
  Bus Selector2 : BusSelector  OutputSignals=robot1MotorParams,robot2MotorParams
  Bus Selector3 : BusSelector  OutputSignals=robot1 calibration params,robot2 calibration params
  Bus to Vector : BusToVector
  Bus to Vector1 : BusToVector
  Create Analog Inputs Subsystem : Subsystem
  Create Custom Data Subsystem : Subsystem
  Create Event Codes Subsystem : Subsystem
  Create KINARM Data Subsystem : Subsystem
  Create Task State Subsystem : Subsystem
  ECAT Status : DataStoreMemory  DataStoreName=ECATStatus  ReadBeforeWriteMsg=error  WriteAfterWriteMsg=warning  WriteAfterReadMsg=error  InitialValue=zeros(1,8)  OutDataTypeStr=double
  ECAT hardware : DataStoreMemory  DataStoreName=ECATHardware  ReadBeforeWriteMsg=error  WriteAfterWriteMsg=warning  WriteAfterReadMsg=error  InitialValue=zeros(1,14)  OutDataTypeStr=double
  Keep alive : Subsystem  TreatAsAtomicUnit=on
      settings: RTWSystemCode=Nonreusable function  RTWFileNameOpts=Use function name
  Memory : Memory
  Memory1 : Memory
  Memory2 : Memory
  Mux : Mux  Inputs=5
  Network Transfer Subsystem : Subsystem  TreatAsAtomicUnit=on
      settings: RTWSystemCode=Nonreusable function  RTWFileNameOpts=Use function name
  Poll Force Plates : Subsystem  TreatAsAtomicUnit=on
      settings: RTWSystemCode=Nonreusable function  RTWFileNameOpts=Use function name
  Poll KINARM : Subsystem  TreatAsAtomicUnit=on
      settings: RTWSystemCode=Nonreusable function  RTWFileNameOpts=Use function name
  Rate Transition : RateTransition
  Rate Transition1 : RateTransition
  Rate Transition2 : RateTransition
  Receive_Gaze : Subsystem  TreatAsAtomicUnit=on
      settings: RTWSystemCode=Nonreusable function  RTWFileNameOpts=Use function name
  Terminators for Gotos : Subsystem
  ZeroDigOut : Constant  Value=[0 0 0 0]
  ZeroEPTorque : Constant  Value=[0 0 0 0]
  ZeroTorque : Constant  Value=[0 0 0 0]
  analog_inputs : Constant  Value=0
  apply loads : Subsystem  TreatAsAtomicUnit=on
      settings: RTWSystemCode=Nonreusable function  RTWFileNameOpts=Use function name
  compare encoders : Subsystem
  read status : DataStoreRead  DataStoreName=ECATStatus  SampleTime=BKIN_STEP_TIME
  tag scope: ECATInitStatus=global, ForcePlateData=global, Gaze_Event_Info=global, Gaze_Global=global, Gaze_pupil_area=global, Gaze_tracking_available=global, KINdata=global, KINdata_bus=global, encoderDeltas=global, has_force_sensor=global, primary_encoder_data=global, primary_encoder_data_bus=global, robot1_calibration_parameters=global, robot1_calibration_parameters_bus=global, robot1_motor_parameters=global, robot2_calibration_parameters=global, robot2_calibration_parameters_bus=global, robot2_motor_parameters=global, status_data=global
  wires:
  ZeroEPTorque/1 -> AddTorques/2
  ZeroTorque/1 -> AddTorques/1
  Bus Selector2/2 -> [robot2_motor_parameters]  "<robot2MotorParams>"
  Bus Selector2/1 -> [robot1_motor_parameters]  "<robot1MotorParams>"
  Bus Selector1/4 -> [primary_encoder_data_bus]  "<primary data bus>"
  Bus Selector1/3 -> [primary_encoder_data]  "<pirmary data>"
  Bus Selector1/2 -> [KINdata_bus]  "<KINDataBus>"
  Bus Selector1/1 -> [KINdata]  "<KINData>"
  Poll KINARM/2(status data) -> [status_data]
  Poll Force Plates/1(force plate data) -> [ForcePlateData]
  Bus Selector/4 -> [Gaze_Event_Info]  "<event info>"
  Bus Selector/3 -> [Gaze_pupil_area]  "<pupil area>"
  Bus Selector/2 -> [Gaze_Global]  "<gaze global>"
  Bus Selector/1 -> [Gaze_tracking_available]  "<gaze available>"
  Rate Transition2/1 -> Mux/2
  Create Custom Data Subsystem/1(Out1) -> Rate Transition/1
  Create Analog Inputs Subsystem/1(Out1) -> Mux/4
  Create KINARM Data Subsystem/1(Out1) -> Mux/3
  Create Event Codes Subsystem/1(Out1) -> Rate Transition2/1
  Create Task State Subsystem/1(Out1) -> Rate Transition1/1
  logging_enable/1 -> Create Task State Subsystem/1(In1)
  Mux/1 -> Network Transfer Subsystem/1(data_frame)
  Rate Transition/1 -> Mux/5
  Rate Transition1/1 -> Mux/1
  Receive_Gaze/1(gaze data) -> [GazeData]
  [GazeData] -> Bus Selector/1
  Poll KINARM/1(kindata) -> [kindata_local]
  [kindata_local] -> Bus Selector1/1
  Poll KINARM/4(robot motor params) -> [motorparams_local]
  [motorparams_local] -> Bus Selector2/1
  [GazeData] -> Poll KINARM/1(gaze data)
  AddTorques/1 -> [torques]
  [torques] -> apply loads/2(torques)
  [torques] -> Memory/1
  Memory/1 -> Poll KINARM/2(torques)
  [motorparams_local] -> Memory2/1
  Poll KINARM/5(sys type) -> [system_type]
  [system_type] -> apply loads/1(system_type)
  Poll KINARM/6(pmac force scale) -> [pmac_force_scale]
  [pmac_force_scale] -> Memory1/1
  Memory1/1 -> apply loads/3(pmac force scale)
  Memory2/1 -> apply loads/4(motor params)
  Poll KINARM/7(robot calibrations) -> [calibration_params_local]
  [calibration_params_local] -> Bus Selector3/1
  Bus Selector3/1 -> [robot1_calibration_parameters_bus], Bus to Vector/1  "<robot1 calibration params>"
  Bus Selector3/2 -> [robot2_calibration_parameters_bus], Bus to Vector1/1  "<robot2 calibration params>"
  Bus to Vector/1 -> [robot1_calibration_parameters]
  Bus to Vector1/1 -> [robot2_calibration_parameters]
  ZeroDigOut/1 -> Poll KINARM/3(digital output)
  compare encoders/1(encoder deltas) -> [encoderDeltas]
  [run_state] -> Poll KINARM/4(run state)
  read status/1 -> [ECATInitStatus]
  event_codes/1 -> Create Event Codes Subsystem/1(In1)
  analog_inputs/1 -> Create Analog Inputs Subsystem/1(In1)
  [global_clock] -> Network Transfer Subsystem/2(global clock)
  [Run_Status] -> Network Transfer Subsystem/3(run_status)
  Poll KINARM/3(hasFT) -> [has_force_sensor]

== system Bruening_4t_showshuffle/KINARM_HandFeedbackInTarget ==
  note: This block was modified from the KINARM_HandInTarget Block to accept cursor position input (i.e. visual
      | representation of hand feedback), rather than the actual position of the hand.
  CursorPos : Inport
  Arm1 : Selector  NumberOfDimensions=2  InputPortWidth=3  IndexOptions=Index vector (dialog),Select all  Indices=1,-1  OutputSizes=slselsubs([(-2),(-2)],1),slselsubs([(-2),(-2)],2)
  Arm2 : Selector  NumberOfDimensions=2  InputPortWidth=3  IndexOptions=Index vector (dialog),Select all  Indices=2,-1  OutputSizes=slselsubs([(-2),(-2)],1),slselsubs([(-2),(-2)],2)
  Array Selector : Selector  NumberOfDimensions=2  InputPortWidth=3  IndexOptions=Select all,Index vector (port)  Indices=-1,1  OutputSizes=slselsubs([(-2),(-2)],1),slselsubs([(-2),(-2)],2)
  Array_Selector1 : Selector  NumberOfDimensions=2  InputPortWidth=3  IndexOptions=Index vector (port),Select all  Indices=-1,1
  Dominant_Arm : Selector  NumberOfDimensions=2  InputPortWidth=3  IndexOptions=Index vector (dialog),Index vector (dialog)  Indices=[3],[1]  OutputSizes=slselsubs([(-2),(-2)],1),slselsubs([(-2),(-2)],2)
  Embedded MATLAB InsideTarget : MATLAB Function  TreatAsAtomicUnit=on
  Embedded MATLAB WhichHand : MATLAB Function  TreatAsAtomicUnit=on
  Hand_Pos : Selector  NumberOfDimensions=2  InputPortWidth=3  IndexOptions=Select all,Index vector (dialog)  Indices=-1,[23,24]  OutputSizes=slselsubs([(-2),(-2)],1),slselsubs([(-2),(-2)],2)
  Multiport Switch : MultiPortSwitch  Inputs=2
  Mux : Mux
  Selected States : Constant  Value=[1]
  Target_Type : Constant  Value=target_type
  Terminator : Terminator
  Use_Dominant_Hand? : Constant  Value=use_dominant_hand
  attribcol1 : Constant  Value=attribcol1
  attribcol2 : Constant  Value=attribcol2
  attribcol3 : Constant  Value=attribcol3
  attribcol4 : Constant  Value=attribcol4
  num_states : Constant  Value=num_states
  HandInTarget_Vector : Outport
  wires:
  Selected States/1 -> Array Selector/2
  num_states/1 -> Embedded MATLAB InsideTarget/4(num_targets)
  Mux/1 -> Embedded MATLAB InsideTarget/3(attribcol)
  attribcol4/1 -> Mux/4
  attribcol3/1 -> Mux/3
  attribcol2/1 -> Mux/2
  attribcol1/1 -> Mux/1
  Use_Dominant_Hand?/1 -> Embedded MATLAB WhichHand/1(use_dominant_hand)
  Embedded MATLAB WhichHand/1(hand) -> Multiport Switch/1
  Target_Type/1 -> Embedded MATLAB InsideTarget/2(target_type)
  Array Selector/1 -> HandInTarget_Vector/1
  [Target_Table] -> Embedded MATLAB InsideTarget/5(Target_Table)
  Embedded MATLAB InsideTarget/1(intarget) -> Array Selector/1
  Multiport Switch/1 -> Terminator/1
  Arm2/1 -> Multiport Switch/3
  Arm1/1 -> Multiport Switch/2
  Dominant_Arm/1 -> Embedded MATLAB WhichHand/2(dominant_hand)
  Hand_Pos/1 -> Arm2/1, Arm1/1
  [KINdata] -> Dominant_Arm/1, Hand_Pos/1
  CursorPos/1 -> Array_Selector1/1
  Array_Selector1/1 -> Embedded MATLAB InsideTarget/1(handpos)
  Embedded MATLAB WhichHand/2(cursor) -> Array_Selector1/2

== system Bruening_4t_showshuffle/Send_Audio_Play ==
  frequency : Inport
  duration : Inport  Port=2
  Trigger : TriggerPort  TriggerType=function-call
  Data Type Conversion : DataTypeConversion  OutDataTypeStr=int32
  Mux : Mux  Inputs=2
  Pack : xpcobsoletelib/Utilities/Pack   datatypes={'int32'}  byteAlign=1
  Send : xpcrtudplib/Legacy UDP/Send   ipAddress=255.255.255.255  ipPort=25255  localPort=-1  vblLen=off  sampletime=-1
  wires:
  Mux/1 -> Pack/1
  Pack/1 -> Send/1
  Data Type Conversion/1 -> Mux/1
  frequency/1 -> Data Type Conversion/1
  duration/1 -> Mux/2
